simulink model "ModelOf3DPrint"  (R2023a)
settings: Solver=ode45  StartTime=0.0  StopTime=100  RelTol=1e-3
settings Model: Creator=ycheb  LastModifiedBy=ycheb

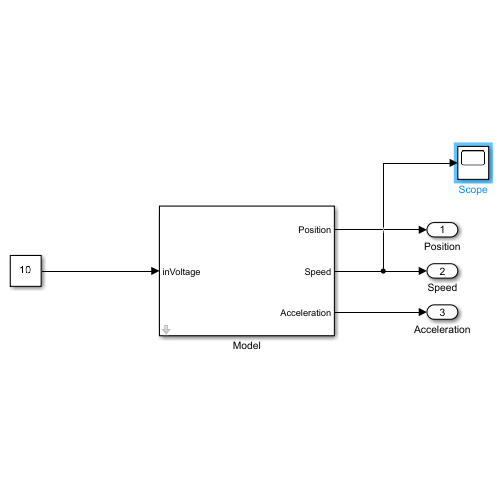
[thumbnail: Simulink's stored preview of the top-level diagram]
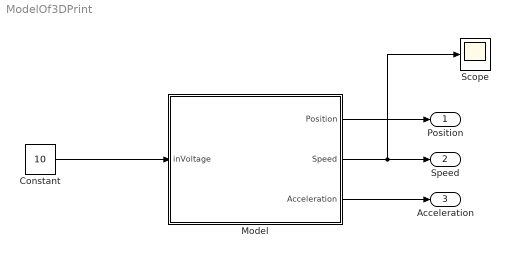
== system ModelOf3DPrint ==
  Constant : Constant  Value=10
  Model : Subsystem  mask{motor_nominal_voltage=24, L=300e-6, R=8.5, km=17e-1, kw=17e-2, J_motor=500e-9, vis_friction_coef_motor=0.001, i_gear=50, J_gear=0.4e-9, vis_friction_coef_gear=0.001, r_wint=0.02, i_wint=12, pen_mass=0.1, vis_friction_coef_pen=0.001, J_wint=0.4e-9}
      mask prompts: motor_nominal_voltage "Motor nominal voltage, V"; L "Rotor inductance, H"; R "Rotor resistance, Ohm"; km "Torgue constant"; kw "Speed constant"; J_motor "Motor inertia, kg*m^2"; vis_friction_coef_motor "Viscous friction coefficient, kg * m^2 / s"; i_gear "Gear aspect ratio"; J_gear "Gear inertia, kg * m^2"; vis_friction_coef_gear "Viscous friction coefficient, kg * m^2 / s"; r_wint "Radius of wint, m"; i_wint "Wint aspect ratio"; pen_mass "Pen mass, kg"; vis_friction_coef_pen "Viscous friction coefficient, kg * m^2 / s"; J_wint "Wint inertia, kg*m^2"
      mask DialogControl Container3 Prompt: Motor Parameters
      mask DialogControl Container4 Prompt: Gear Paremeters
      mask DialogControl Container5 Prompt: Wint parameters
  Scope : Scope
  Position : Outport
  Speed : Outport  Port=2
  Acceleration : Outport  Port=3
  wires:
  Constant/1 -> Model/1(inVoltage)
  Model/1(Position) -> Position/1
  Model/2(Speed) -> Scope/1, Speed/1
  Model/3(Acceleration) -> Acceleration/1

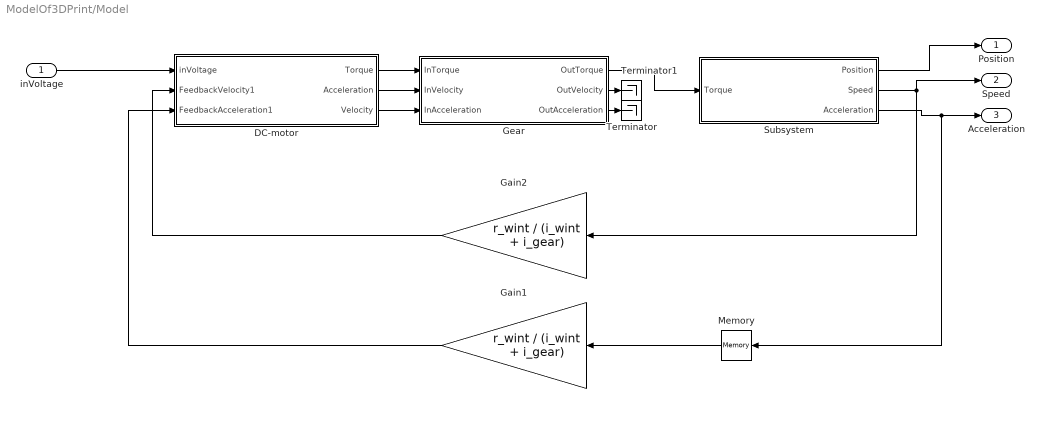
== system ModelOf3DPrint/Model ==
  inVoltage : Inport
  DC-motor : Subsystem  TreatAsAtomicUnit=on
      settings: RTWFcnNameOpts=Use subsystem name  RTWFileNameOpts=Use function name
  Gain1 : Gain  Gain=r_wint / (i_wint + i_gear)
  Gain2 : Gain  Gain=r_wint / (i_wint + i_gear)
  Gear : Subsystem
  Memory : Memory
  Subsystem : Subsystem
  Terminator : Terminator
  Terminator1 : Terminator
  Position : Outport
  Speed : Outport  Port=2
  Acceleration : Outport  Port=3
  wires:
  Gear/2(OutVelocity) -> Terminator1/1
  Subsystem/1(Position) -> Position/1
  DC-motor/1(Torque) -> Gear/1(InTorque)
  DC-motor/3(Velocity) -> Gear/3(InAcceleration)
  Subsystem/3(Acceleration) -> Acceleration/1, Memory/1
  inVoltage/1 -> DC-motor/1(inVoltage)
  Gear/1(OutTorque) -> Subsystem/1(Torque)
  Subsystem/2(Speed) -> Speed/1, Gain2/1
  Gear/3(OutAcceleration) -> Terminator/1
  DC-motor/2(Acceleration) -> Gear/2(InVelocity)
  Gain1/1 -> DC-motor/3(FeedbackAcceleration1)
  Gain2/1 -> DC-motor/2(FeedbackVelocity1)
  Memory/1 -> Gain1/1

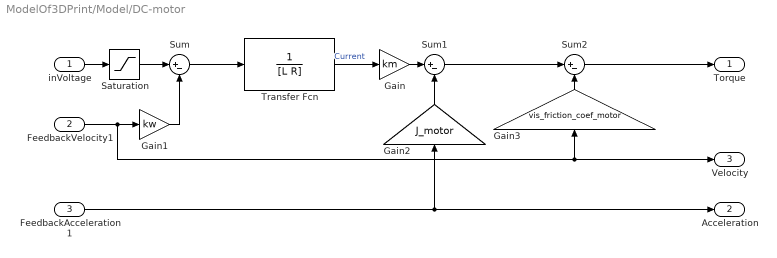
== system ModelOf3DPrint/Model/DC-motor ==
  inVoltage : Inport
  FeedbackVelocity1 : Inport  Port=2
  FeedbackAcceleration1 : Inport  Port=3
  Gain : Gain  Gain=km
  Gain1 : Gain  Gain=kw
  Gain2 : Gain  Gain=J_motor
  Gain3 : Gain  Gain=vis_friction_coef_motor
  Saturation : Saturate  UpperLimit=motor_nominal_voltage  LowerLimit=-motor_nominal_voltage
  Sum : Sum  Inputs=|+-
  Sum1 : Sum  Inputs=|+-
  Sum2 : Sum  Inputs=|+-
  Transfer Fcn : TransferFcn  Denominator=[L R]
  Torque : Outport
  Acceleration : Outport  Port=2
  Velocity : Outport  Port=3
  wires:
  Sum1/1 -> Sum2/1
  FeedbackVelocity1/1 -> Velocity/1, Gain3/1, Gain1/1
  Gain2/1 -> Sum1/2
  Gain1/1 -> Sum/2
  Sum/1 -> Transfer Fcn/1
  Gain3/1 -> Sum2/2
  Transfer Fcn/1 -> Gain/1  "Current"
  inVoltage/1 -> Saturation/1
  Gain/1 -> Sum1/1
  FeedbackAcceleration1/1 -> Acceleration/1, Gain2/1
  Sum2/1 -> Torque/1
  Saturation/1 -> Sum/1

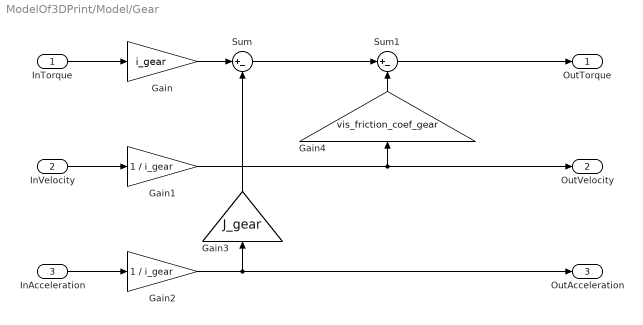
== system ModelOf3DPrint/Model/Gear ==
  InTorque : Inport
  InVelocity : Inport  Port=2
  InAcceleration : Inport  Port=3
  Gain : Gain  Gain=i_gear
  Gain1 : Gain  Gain=1 / i_gear
  Gain2 : Gain  Gain=1 / i_gear
  Gain3 : Gain  Gain=J_gear
  Gain4 : Gain  Gain=vis_friction_coef_gear
  Sum : Sum  Inputs=|+-
  Sum1 : Sum  Inputs=|+-
  OutTorque : Outport
  OutVelocity : Outport  Port=2
  OutAcceleration : Outport  Port=3
  wires:
  Sum1/1 -> OutTorque/1
  Gain3/1 -> Sum/2
  Gain4/1 -> Sum1/2
  Sum/1 -> Sum1/1
  InTorque/1 -> Gain/1
  Gain/1 -> Sum/1
  InAcceleration/1 -> Gain2/1
  InVelocity/1 -> Gain1/1
  Gain2/1 -> Gain3/1, OutAcceleration/1
  Gain1/1 -> Gain4/1, OutVelocity/1

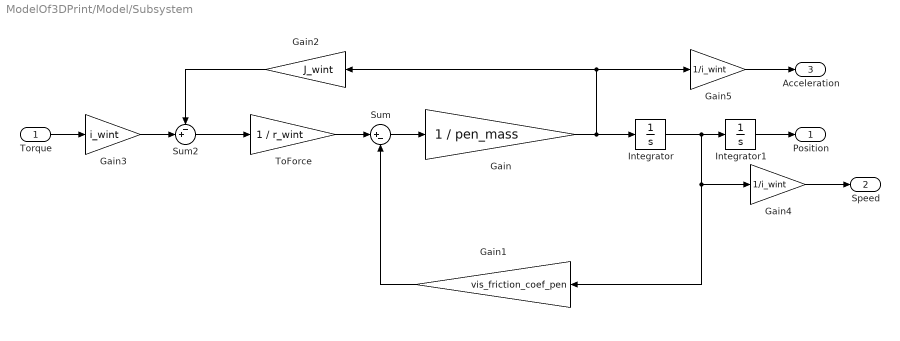
== system ModelOf3DPrint/Model/Subsystem ==
  Torque : Inport
  Gain : Gain  Gain=1 / pen_mass
  Gain1 : Gain  Gain=vis_friction_coef_pen
  Gain2 : Gain  Gain=J_wint
  Gain3 : Gain  Gain=i_wint
  Gain4 : Gain  Gain=1/i_wint
  Gain5 : Gain  Gain=1/i_wint
  Integrator : Integrator
  Integrator1 : Integrator
  Sum : Sum  Inputs=|+-
  Sum2 : Sum  Inputs=-+|
  ToForce : Gain  Gain=1 / r_wint
  Position : Outport
  Speed : Outport  Port=2
  Acceleration : Outport  Port=3
  wires:
  Gain2/1 -> Sum2/1
  Gain/1 -> Integrator/1, Gain5/1, Gain2/1
  Sum2/1 -> ToForce/1
  Torque/1 -> Gain3/1
  ToForce/1 -> Sum/1
  Sum/1 -> Gain/1
  Integrator/1 -> Gain4/1, Gain1/1, Integrator1/1
  Integrator1/1 -> Position/1
  Gain1/1 -> Sum/2
  Gain3/1 -> Sum2/2
  Gain4/1 -> Speed/1
  Gain5/1 -> Acceleration/1
